simulink model "NE39bus2_PQ"  (R2023b)
settings: Solver=ode23tb  StartTime=0.0  StopTime=120  MaxStep=1/60  RelTol=1e-2  AbsTol=1e-1  EnableMultiTasking=on
PreLoadFcn:
  | NE39bus_data;
  | PSSMODEL=1;
  | LPSS=0;
  | WAPSS=0;
  | WAPSS2=0;
values from neighbouring files (symbols this model uses):
  AVR_Data = [     0.01  200    0.015   10    1    1.03    -5    5 ... (first row only)    [NE39bus_data.m]
  line = [     1	2	0.0035	0.0411	0.6987	0	100	345 ... (first row only)    [NE39bus_data.m]
  mac_con = [ ... (first row only)    [NE39bus_data.m]
  MB = [1   0.2 30   1.25 40    12 160]    [NE39bus_data.m]
  Ns = 120*60/(2)    (= 3600)    [NE39bus_data.m]
  p0 = [1000 520.81 650 632 508 650 560 540 830 250]'./1000    [NE39bus_data.m]
  s = 10    [NE39bus_data.m]
undefined symbols (not defined in the file or in its folder): D1, Delta, Pn
libraries: spsThreePhaseVIMeasurementLib x56, spsThreePhasePISectionLineLib x38, spsGenericPowerSystemStabilizerLib x20, spsThreePhaseParallelRLCLoadLib x19, spsThreePhaseTransformerTwoWindingsLib x16, spsSynchronousMachinepuStandardLib x10, spsExcitationSystemLib x10, spsMultiBandPowerSystemStabilizerLib x10, spsSteamTurbineandGovernorLib x10, spsLoadFlowBusLib x10, powerlib_extras x4, spsThreePhaseDynamicLoadLib x4
(part 4 of 5)

== system NE39bus2_PQ/G8/M8: Turbine & Regulators ==
  note: M8
  m8 : Inport
  Pref8 : Inport  Port=2
  Vref8 : Inport  Port=3
  PSS8 : Inport  Port=4
  Bus Selector : BusSelector  OutputSignals="Mechanical.Rotor speed  wm  (pu),Mechanical.Rotor angle deviation  d_theta (rad),Mechanical.Electrical power  Pe (pu),Mechanical.Rotor speed deviation  dw (pu),Mechanical.Rotor mechanical angle  theta (deg),dq0 components.Stator voltage  vd (pu),dq0 components.Stator voltage  vq (pu),Output reactive power  Qeo (pu)"
  Delta Pa PSS 8 : spsGenericPowerSystemStabilizerLib/Generic Power System Stabilizer  Tsensor=15e-3  K=2.5*1.25  Twashout=1  Tleadlag1=[60e-3 1]  Tleadlag2=[0 0]  VSlimits=[-0.15 0.15]  Vinit=0  Plot_On=off  MagdB_On=on  FreqRange=logspace(-2,2,500)
      settings: LibrarySourceBlock=|
      | sps_lib/Electrical Machines/Synchronous Machine Control/Generic
      | Power System Stabilizer
  Delta w PSS (Kundur) 8 : spsGenericPowerSystemStabilizerLib/Generic Power System Stabilizer  Tsensor=15e-3  K=30  Twashout=10  Tleadlag1=[50e-3 20e-3]  Tleadlag2=[3 5.4]  VSlimits=[-0.15 0.15]  Vinit=0  Plot_On=off  MagdB_On=on  FreqRange=logspace(-2,2,500)
      settings: LibrarySourceBlock=|
      | sps_lib/Electrical Machines/Synchronous Machine Control/Generic
      | Power System Stabilizer
  EXCITATION8 : spsExcitationSystemLib/Excitation System  tr=AVR_Data(8,1)  reg=[ AVR_Data(8,2:3) ]  exc=[ 1, 0 ]  tgr=[ AVR_Data(8,4:5)]  damp=[ 0, 0 ]  sat=[ 0, 0 ]  lim="[ AVR_Data(8,7:8)  0 ]"  v0=[1,1.90805]
      settings: LibrarySourceBlock=sps_lib/Electrical Machines/Synchronous Machine Control/Excitation System
  MB-PSS8 : spsMultiBandPowerSystemStabilizerLib/Multi-Band Power System Stabilizer  OperationMode=Simplified settings  Kg=MB(1)  GL=[MB(2) MB(3)]  GI=[MB(4) MB(5)]  GH=[MB(6) MB(7)]  GLd=[66 66 9.4]  TcLF=[1.667 2 0 0 0 0 2 2.4 0 0 0 0 1 1]  GId=[66 66 47.6]  TcIF=[1 1 0.25 0.3 0 0 1 1 0.3 0.36 0 0 0 0]  GHd=[66 66 233]  TcHF="[0.01 0.012 0 0 0 0  0.012 0.0144 0 0 0 0 1 1]"  LIM=[.075 .15 .15 .15]  Plot_On=off  MagdB_On=off  FreqRange=logspace(-2,2,500)
      settings: LibrarySourceBlock=|
      | sps_lib/Electrical Machines/Synchronous Machine Control/Multi-Band
      | Power System Stabilizer
  Multiport Switch2 : MultiPortSwitch  Inputs=4  SaturateOnIntegerOverflow=off
  PSS model1 : Constant  Value=0
  PSS model2 : Constant
  Real-Imag to Complex1 : RealImagToComplex
  STG8 : spsSteamTurbineandGovernorLib/Steam Turbine and Governor  gentype=Tandem-compound (single mass)  reg1="[ 1  0.05    0 ]"  reg2="[ 0.001  0.15 ]"  reg3="[ -0.1  0.1  0  4.496 ]"  N=Ns  turb1="[ 0  10   3.3   0.5   ]"  turb2="[   0   0.36    0.36   0.28   ]"  HA="[ 0.046  1.430  1.465   0.192 ]"  KA="[ 90.44  53.88  64.59   62.94  ]"  DA="[ 0.0115  0.3575  0.3663   0.0137  ]"  ini1=0.54  ini2=[0.779316,-31.4247]
      settings: LibrarySourceBlock=|
      | sps_lib/Electrical Machines/Synchronous Machine Control/Steam Turbine
      | and Governor
  Sum1 : Sum  Inputs=-+  InputSameDT=on  SaturateOnIntegerOverflow=on  OutDataTypeStr=Inherit: Same as first input
  Sum2 : Sum  InputSameDT=on  SaturateOnIntegerOverflow=on  OutDataTypeStr=Inherit: Same as first input
  Terminator3 : Terminator
  Terminator4 : Terminator
  Terminator5 : Terminator
  wref8 : Constant
  Pm8 : Outport  InitialOutput=0
  Vf8 : Outport  Port=2  InitialOutput=0
  tag scope: EFD8=global, Pa8=global, Pe8=global, Q8=global, Vt8=global, d_theta8=global, pss8=global, theta8=global, w8=global
  wires:
  Bus Selector/7 -> EXCITATION8/3, Real-Imag to Complex1/2  "<Stator voltage  vq (pu)>"
  wref8/1 -> STG8/1
  Pref8/1 -> STG8/2
  m8/1 -> Bus Selector/1
  Vref8/1 -> EXCITATION8/1
  EXCITATION8/1 -> Vf8/1, [EFD8]
  Real-Imag to Complex1/1 -> [Vt8]
  Bus Selector/5 -> [theta8]  "<Rotor mechanical angle  theta (deg)>"
  Bus Selector/6 -> EXCITATION8/2, Real-Imag to Complex1/1  "<Stator voltage  vd (pu)>"
  STG8/3 -> Terminator3/1
  STG8/4 -> Sum1/2, Pm8/1
  STG8/2 -> Terminator4/1
  STG8/1 -> Terminator5/1
  Bus Selector/1 -> [w8], STG8/3  "<Rotor speed  wm  (pu)>"
  Bus Selector/2 -> STG8/4, [d_theta8]  "<Rotor angle deviation  d_theta (rad)>"
  Bus Selector/3 -> Sum1/1, [Pe8]  "<Electrical power  Pe (pu)>"
  Bus Selector/4 -> MB-PSS8/1, Delta w PSS (Kundur) 8/1  "<Rotor speed deviation  dw (pu)>"
  Bus Selector/8 -> [Q8]  "<Output reactive power  Qeo (pu)>"
  Sum1/1 -> [Pa8], Delta Pa PSS 8/1  "Pm-Pe"
  Sum2/1 -> Multiport Switch2/1
  PSS model2/1 -> Sum2/2
  Delta Pa PSS 8/1 -> Multiport Switch2/5
  Delta w PSS (Kundur) 8/1 -> Multiport Switch2/4
  MB-PSS8/1 -> Multiport Switch2/3
  PSS model1/1 -> Multiport Switch2/2
  Multiport Switch2/1 -> EXCITATION8/4, [pss8]
  PSS8/1 -> Sum2/1

== system NE39bus2_PQ/G9/M9: Turbine & Regulators  ==
  note: M9
  m9 : Inport
  Pref9 : Inport  Port=2
  Vref9 : Inport  Port=3
  PSS9 : Inport  Port=4
  Bus Selector : BusSelector  OutputSignals="Mechanical.Rotor speed  wm  (pu),Mechanical.Rotor angle deviation  d_theta (rad),Mechanical.Electrical power  Pe (pu),Mechanical.Rotor speed deviation  dw (pu),Mechanical.Rotor mechanical angle  theta (deg),dq0 components.Stator voltage  vd (pu),dq0 components.Stator voltage  vq (pu),Output reactive power  Qeo (pu)"
  Delta Pa PSS 9 : spsGenericPowerSystemStabilizerLib/Generic Power System Stabilizer  Tsensor=15e-3  K=2.5*1.25  Twashout=1  Tleadlag1=[60e-3 1]  Tleadlag2=[0 0]  VSlimits=[-0.15 0.15]  Vinit=0  Plot_On=off  MagdB_On=on  FreqRange=logspace(-2,2,500)
      settings: LibrarySourceBlock=|
      | sps_lib/Electrical Machines/Synchronous Machine Control/Generic
      | Power System Stabilizer
  Delta w PSS (Kundur) 9 : spsGenericPowerSystemStabilizerLib/Generic Power System Stabilizer  Tsensor=15e-3  K=30  Twashout=10  Tleadlag1=[50e-3 20e-3]  Tleadlag2=[3 5.4]  VSlimits=[-0.15 0.15]  Vinit=0  Plot_On=off  MagdB_On=on  FreqRange=logspace(-2,2,500)
      settings: LibrarySourceBlock=|
      | sps_lib/Electrical Machines/Synchronous Machine Control/Generic
      | Power System Stabilizer
  EXCITATION9 : spsExcitationSystemLib/Excitation System  tr=AVR_Data(9,1)  reg=[ AVR_Data(9,2:3) ]  exc=[ 1, 0 ]  tgr=[ AVR_Data(9,4:5)]  damp=[ 0, 0 ]  sat=[ 0, 0 ]  lim="[ AVR_Data(9,7:8)  0 ]"  v0=[1,2.08155]
      settings: LibrarySourceBlock=sps_lib/Electrical Machines/Synchronous Machine Control/Excitation System
  MB-PSS9 : spsMultiBandPowerSystemStabilizerLib/Multi-Band Power System Stabilizer  OperationMode=Simplified settings  Kg=MB(1)  GL=[MB(2) MB(3)]  GI=[MB(4) MB(5)]  GH=[MB(6) MB(7)]  GLd=[66 66 9.4]  TcLF=[1.667 2 0 0 0 0 2 2.4 0 0 0 0 1 1]  GId=[66 66 47.6]  TcIF=[1 1 0.25 0.3 0 0 1 1 0.3 0.36 0 0 0 0]  GHd=[66 66 233]  TcHF="[0.01 0.012 0 0 0 0  0.012 0.0144 0 0 0 0 1 1]"  LIM=[.075 .15 .15 .15]  Plot_On=off  MagdB_On=off  FreqRange=logspace(-2,2,500)
      settings: LibrarySourceBlock=|
      | sps_lib/Electrical Machines/Synchronous Machine Control/Multi-Band
      | Power System Stabilizer
  Multiport Switch1 : MultiPortSwitch  Inputs=4  SaturateOnIntegerOverflow=off
  PSS model3 : Constant  Value=0
  PSS model4 : Constant
  Real-Imag to Complex1 : RealImagToComplex
  STG9 : spsSteamTurbineandGovernorLib/Steam Turbine and Governor  gentype=Tandem-compound (single mass)  reg1="[ 1  0.05    0 ]"  reg2="[ 0.001  0.15 ]"  reg3="[ -0.1  0.1  0  4.496 ]"  N=Ns  turb1="[ 0  10   3.3   0.5   ]"  turb2="[   0   0.36    0.36   0.28   ]"  HA="[ 0.046  1.430  1.465   0.192 ]"  KA="[ 90.44  53.88  64.59   62.94  ]"  DA="[ 0.0115  0.3575  0.3663   0.0137  ]"  ini1=0.83  ini2=[0.779316,-31.4247]
      settings: LibrarySourceBlock=|
      | sps_lib/Electrical Machines/Synchronous Machine Control/Steam Turbine
      | and Governor
  Sum2 : Sum  InputSameDT=on  SaturateOnIntegerOverflow=on  OutDataTypeStr=Inherit: Same as first input
  Sum3 : Sum  Inputs=-+  InputSameDT=on  SaturateOnIntegerOverflow=on  OutDataTypeStr=Inherit: Same as first input
  Terminator3 : Terminator
  Terminator4 : Terminator
  Terminator5 : Terminator
  wref9 : Constant
  Pm9 : Outport  InitialOutput=0
  Vf9 : Outport  Port=2  InitialOutput=0
  tag scope: EFD9=global, Pa9=global, Pe9=global, Q9=global, Vt9=global, d_theta9=global, pss9=global, theta9=global, w9=global
  wires:
  Bus Selector/7 -> EXCITATION9/3, Real-Imag to Complex1/2  "<Stator voltage  vq (pu)>"
  wref9/1 -> STG9/1
  Pref9/1 -> STG9/2
  m9/1 -> Bus Selector/1
  Vref9/1 -> EXCITATION9/1
  EXCITATION9/1 -> Vf9/1, [EFD9]
  Real-Imag to Complex1/1 -> [Vt9]
  Bus Selector/5 -> [theta9]  "<Rotor mechanical angle  theta (deg)>"
  Bus Selector/6 -> EXCITATION9/2, Real-Imag to Complex1/1  "<Stator voltage  vd (pu)>"
  STG9/3 -> Terminator3/1
  STG9/4 -> Sum3/2, Pm9/1
  STG9/2 -> Terminator4/1
  STG9/1 -> Terminator5/1
  Bus Selector/1 -> [w9], STG9/3  "<Rotor speed  wm  (pu)>"
  Bus Selector/2 -> STG9/4, [d_theta9]  "<Rotor angle deviation  d_theta (rad)>"
  Bus Selector/3 -> Sum3/1, [Pe9]  "<Electrical power  Pe (pu)>"
  Bus Selector/4 -> Delta w PSS (Kundur) 9/1, MB-PSS9/1  "<Rotor speed deviation  dw (pu)>"
  Bus Selector/8 -> [Q9]  "<Output reactive power  Qeo (pu)>"
  Sum3/1 -> [Pa9], Delta Pa PSS 9/1  "Pm-Pe"
  Sum2/1 -> Multiport Switch1/1
  PSS model4/1 -> Sum2/2
  Delta Pa PSS 9/1 -> Multiport Switch1/5
  Delta w PSS (Kundur) 9/1 -> Multiport Switch1/4
  MB-PSS9/1 -> Multiport Switch1/3
  PSS model3/1 -> Multiport Switch1/2
  Multiport Switch1/1 -> [pss9], EXCITATION9/4
  PSS9/1 -> Sum2/1

== matlab function NE39bus2_PQ/DCLoad3/DC Composite Model/DC ==
  data: V_pu input; P_out output; Q_out output; t input; ups_state output; cool_stall output; P_it_out output; P_ai_pu input; P_cool_out output; Pdc_MW input
function [P_out, Q_out, ups_state, cool_stall, P_it_out, P_cool_out] = ...
    datacenter_motorE(V_pu, t, P_ai_pu, Pdc_MW)
%#codegen
% =========================================================================
% WECC CLM Extension: Data Center Load Model (Motor E)
% Scalable from 100 MW to 500 MW
% =========================================================================
% Inputs:  V_pu    = per-unit voltage at load bus
%          t       = simulation time
%          P_ai_pu = AI workload demand (0-1 pu)
%          Pdc_MW  = data center rated power in MW (100 to 500)
%
% Outputs: P_out (W), Q_out (VAR)
%          ups_state, cool_stall, P_it_out, P_cool_out
%
% Block sample time = 0.001
% =========================================================================

dt = 0.001;

% ===== DATA CENTER SIZING =====
Pdc = double(Pdc_MW(1)) * 1e6;    % convert MW to W

% ===== SUB-COMPONENT FRACTIONS =====
% Based on industry data:
% IT load (servers/GPUs): 55-65% -> 60%
% Cooling (chillers/CRAH): 25-35% -> 30%
% Auxiliary (lighting/office/network): 8-12% -> 10%
Fit_max  = 0.60;
Fcool    = 0.30;
Faux     = 0.10;

% ===== UPS PARAMETERS =====
% Large DC UPS: tighter voltage tolerance, faster transfer
V_ups_trip    = 0.90;    % static transfer switch threshold
V_ups_return  = 0.95;    % return to grid threshold
T_ups_battery = 30.0;    % battery hold-up time (s)
T_diesel_start = 12.0;   % diesel generator start time (s)
T_ups_transfer = 0.004;  % static switch transfer time (s)
PF_it = 0.95;

% ===== COOLING PARAMETERS =====
% Industrial chillers: higher inertia, different stall characteristics
Rstall_c = 0.10;     Xstall_c = 0.12;
Vstall_c = 0.55;     % industrial compressors stall lower than residential
Tstall_c = 0.05;     % stall confirmation delay
Vrst_c   = 0.90;     Trst_c = 2.0;   % slower restart (large chillers)
TTH_c    = 60;        % higher thermal mass (industrial)
th1_c    = 1.6;       th2_c = 2.8;    % wider thermal margin
PF_cool  = 0.85;

% ===== VFD COOLING FRACTION =====
% Modern DCs use VFDs on some chillers (don't stall, ride through)
Fvfd = 0.40;    % 40% of cooling on VFDs (constant power during fault)

% ===== PERSISTENT STATE =====
persistent ups_mode batt_timer diesel_timer transfer_cnt
persistent is_cool_stalled cool_stall_cnt cool_rst_cnt
persistent theta_cool fth_cool
persistent P_it_before_fault
persistent rebound_active rebound_timer
persistent init_done

if isempty(init_done)
    ups_mode          = 0;
    batt_timer        = 0;
    diesel_timer      = 0;
    transfer_cnt      = 0;
    is_cool_stalled   = false;
    cool_stall_cnt    = 0;
    cool_rst_cnt      = 0;
    theta_cool        = 0;
    fth_cool          = 1;
    P_it_before_fault = 0;
    rebound_active    = false;
    rebound_timer     = 0;
    init_done         = true;
end

% Soft start
if t < 1.0
    ramp = t / 1.0;
    P_out = Pdc * 0.7 * ramp;
    Q_out = Pdc * 0.25 * ramp;
    ups_state  = 0;
    cool_stall = 0;
    P_it_out   = Fit_max * Pdc * 0.9 * ramp;
    P_cool_out = Fcool * Pdc * ramp;
    return;
end

V = double(V_pu(1));
if V < 0.01
    V = 0.01;
end
if V > 1.5
    V = 1.5;
end

P_ai = double(P_ai_pu(1));
if P_ai < 0.05
    P_ai = 0.05;
end
if P_ai > 1.0
    P_ai = 1.0;
end

% =========================================================
% COMPONENT 1: IT LOAD WITH UPS + AI WORKLOAD
% =========================================================
P_it_demand = Fit_max * Pdc * P_ai;
Q_it_demand = P_it_demand * tan(acos(PF_it));

P_it = 0;
Q_it = 0;

if ups_mode == 0
    % GRID-CONNECTED: IT load on grid, scaled by workload
    P_it_before_fault = P_it_demand;
    
    if V < V_ups_trip
        ups_mode = 1;
        batt_timer = 0;
        diesel_timer = 0;
        transfer_cnt = 0;
    end
    
    P_it = P_it_demand;
    Q_it = Q_it_demand;
    
elseif ups_mode == 1
    % UPS BATTERY MODE: IT load invisible to grid
    batt_timer = batt_timer + dt;
    diesel_timer = diesel_timer + dt;
    transfer_cnt = transfer_cnt + dt;
    
    if transfer_cnt < T_ups_transfer
        % During transfer: partial load visible
        P_it = P_it_before_fault * 0.3;
        Q_it = Q_it_demand * 0.3;
    else
        % Fully on battery: zero grid draw
        P_it = 0;
        Q_it = 0;
    end
    
    if V >= V_ups_return
        % Voltage recovered: LOAD REBOUND
        ups_mode = 0;
        rebound_active = true;
        rebound_timer = 0;
        batt_timer = 0;
    elseif diesel_timer >= T_diesel_start
        ups_mode = 2;
    elseif batt_timer >= T_ups_battery
        ups_mode = 0;  % forced return
        rebound_active = true;
        rebound_timer = 0;
    end
    
elseif ups_mode == 2
    % DIESEL BACKUP: permanently off grid
    P_it = 0;
    Q_it = 0;
end

% LOAD REBOUND: IT load returns to grid with inrush
% Causes a secondary voltage dip
if rebound_active
    rebound_timer = rebound_timer + dt;
    rebound_duration = 0.5;  % 500ms rebound transient
    
    if rebound_timer < rebound_duration
        % During rebound: 120% of pre-fault load (inrush)
        rebound_factor = 1.2 - 0.2 * (rebound_timer / rebound_duration);
        P_it = P_it * rebound_factor;
        Q_it = Q_it * rebound_factor * 1.5;  % higher Q during rebound
    else
        rebound_active = false;
    end
end

% =========================================================
% COMPONENT 2: COOLING LOAD (split: motor + VFD)
% =========================================================

Zstall_sq = Rstall_c * Rstall_c + Xstall_c * Xstall_c;
Gstall_cool = Rstall_c / Zstall_sq;
Bstall_cool = Xstall_c / Zstall_sq;

% Cooling demand proportional to IT workload
cool_scale = 0.4 + 0.6 * P_ai;  % 60-100% cooling

P_cool_base = Fcool * Pdc * cool_scale;
Q_cool_base = P_cool_base * tan(acos(PF_cool));

% --- Motor-driven portion (1-Fvfd): can stall ---
P_motor_rated = (1.0 - Fvfd) * P_cool_base;
Q_motor_rated = (1.0 - Fvfd) * Q_cool_base;

P_motor_stall = Gstall_cool * V * V * (1.0 - Fvfd) * Fcool * Pdc;
Q_motor_stall = -Bstall_cool * V * V * (1.0 - Fvfd) * Fcool * Pdc;

% Stall logic (motor portion only)
if ~is_cool_stalled
    if V < Vstall_c
        cool_stall_cnt = cool_stall_cnt + dt;
        if cool_stall_cnt >= Tstall_c
            is_cool_stalled = true;
            cool_stall_cnt = 0;
        end
    else
        cool_stall_cnt = 0;
    end
else
    if V >= Vrst_c
        cool_rst_cnt = cool_rst_cnt + dt;
        if cool_rst_cnt >= Trst_c
            is_cool_stalled = false;
            cool_rst_cnt = 0;
            theta_cool = 0;
        end
    else
        cool_rst_cnt = 0;
    end
end

% Thermal relay
if is_cool_stalled
    I_sq = V * V / Zstall_sq;
    theta_cool = theta_cool + (I_sq * Rstall_c - theta_cool) / TTH_c * dt;
    if theta_cool < 0
        theta_cool = 0;
    end
    if theta_cool >= th2_c
        fth_cool = 0;
    elseif theta_cool >= th1_c
        fth_cool = 1.0 - (theta_cool - th1_c) / (th2_c - th1_c);
        if fth_cool < 0
            fth_cool = 0;
        end
    else
        fth_cool = 1.0;
    end
else
    if theta_cool > 0.001
        theta_cool = theta_cool * (1.0 - dt / TTH_c);
    else
        theta_cool = 0;
    end
    fth_cool = 1.0;
end

% Motor cooling output
if is_cool_stalled
    P_motor = P_motor_stall * fth_cool;
    Q_motor = Q_motor_stall * fth_cool;
else
    P_motor = P_motor_rated * V * V;
    Q_motor = Q_motor_rated * V * V;
end

% --- VFD portion (Fvfd): rides through, constant power ---
% VFDs maintain constant power down to ~0.5 pu voltage
if V >= 0.5
    P_vfd = Fvfd * P_cool_base;
    Q_vfd = Fvfd * Q_cool_base * 0.5;  % VFDs have lower Q
elseif V >= 0.3
    % Linear reduction below 0.5
    vfd_frac = (V - 0.3) / 0.2;
    P_vfd = Fvfd * P_cool_base * vfd_frac;
    Q_vfd = Fvfd * Q_cool_base * 0.5 * vfd_frac;
else
    P_vfd = 0;
    Q_vfd = 0;
end

P_cool = P_motor + P_vfd;
Q_cool = Q_motor + Q_vfd;

% =========================================================
% COMPONENT 3: AUXILIARY (constant impedance)
% =========================================================
P_aux = Faux * Pdc * V * V;
Q_aux = Faux * Pdc * 0.15 * V * V;

% =========================================================
% TOTAL DATA CENTER OUTPUT
% =========================================================
P_out = P_it + P_cool + P_aux;
Q_out = Q_it + Q_cool + Q_aux;

if P_out < 0
    P_out = 0;
end

ups_state = double(ups_mode);
if is_cool_stalled
    cool_stall = 1.0;
else
    cool_stall = 0.0;
end
P_it_out = P_it;
P_cool_out = P_cool;

end

== matlab function NE39bus2_PQ/DCLoad1/DC Composite Model/AI Workload Generator ==
  data: t input; mode input; P_ai_pu output; workload_label output
function [P_ai_pu, workload_label] = ai_workload(t, mode)
%#codegen
% AI GPU Workload Profile Generator
% mode: 1=Training, 2=Inference, 3=Idle
% Output: P_ai_pu (0 to 1), workload_label

workload_label = double(mode);

if mode == 1
    % TRAINING: sustained high with checkpoint dips
    base_power = 0.3;
    checkpoint_interval = 60.0;
    checkpoint_duration = 2.0;
    checkpoint_dip = 0.40;
    comm_period = 1.2;
    comm_amplitude = 0.6;
    
    time_in_cycle = mod(t, checkpoint_interval);
    if time_in_cycle < checkpoint_duration
        P_ai_pu = checkpoint_dip;
    else
        oscillation = comm_amplitude * sin(2.0 * 3.14159 * t / comm_period);
        P_ai_pu = base_power + oscillation;
    end
    
elseif mode == 2
    % INFERENCE: bursty multi-frequency
    base_power = 0.15;
    burst1 = 0.25 * sin(2.0 * 3.14159 * t / 5.0);
    burst2 = 0.15 * sin(2.0 * 3.14159 * t / 1.3);
    burst3 = 0.10 * sin(2.0 * 3.14159 * t / 0.4);
    
    if t < 2.0
        diurnal = 0.5 + 0.5 * (t / 2.0);
    else
        diurnal = 1.0;
    end
    
    P_ai_pu = (base_power + burst1 + burst2 + burst3) * diurnal;
    
elseif mode == 3
    % IDLE
    P_ai_pu = 0.15;
else
    P_ai_pu = 0.5;
end

if P_ai_pu < 0.05
    P_ai_pu = 0.05;
end
if P_ai_pu > 1.0
    P_ai_pu = 1.0;
end

end

== matlab function NE39bus2_PQ/DCLoad1/DC Composite Model/DC ==
  data: V_pu input; P_out output; Q_out output; t input; ups_state output; cool_stall output; P_it_out output; P_ai_pu input; P_cool_out output; Pdc_MW input
function [P_out, Q_out, ups_state, cool_stall, P_it_out, P_cool_out] = ...
    datacenter_motorE(V_pu, t, P_ai_pu, Pdc_MW)
%#codegen
% =========================================================================
% WECC CLM Extension: Data Center Load Model (Motor E)
% Scalable from 100 MW to 500 MW
% =========================================================================
% Inputs:  V_pu    = per-unit voltage at load bus
%          t       = simulation time
%          P_ai_pu = AI workload demand (0-1 pu)
%          Pdc_MW  = data center rated power in MW (100 to 500)
%
% Outputs: P_out (W), Q_out (VAR)
%          ups_state, cool_stall, P_it_out, P_cool_out
%
% Block sample time = 0.001
% =========================================================================

dt = 0.001;

% ===== DATA CENTER SIZING =====
Pdc = double(Pdc_MW(1)) * 1e6;    % convert MW to W

% ===== SUB-COMPONENT FRACTIONS =====
% Based on industry data:
% IT load (servers/GPUs): 55-65% -> 60%
% Cooling (chillers/CRAH): 25-35% -> 30%
% Auxiliary (lighting/office/network): 8-12% -> 10%
Fit_max  = 0.60;
Fcool    = 0.30;
Faux     = 0.10;

% ===== UPS PARAMETERS =====
% Large DC UPS: tighter voltage tolerance, faster transfer
V_ups_trip    = 0.90;    % static transfer switch threshold
V_ups_return  = 0.95;    % return to grid threshold
T_ups_battery = 30.0;    % battery hold-up time (s)
T_diesel_start = 12.0;   % diesel generator start time (s)
T_ups_transfer = 0.004;  % static switch transfer time (s)
PF_it = 0.95;

% ===== COOLING PARAMETERS =====
% Industrial chillers: higher inertia, different stall characteristics
Rstall_c = 0.10;     Xstall_c = 0.12;
Vstall_c = 0.55;     % industrial compressors stall lower than residential
Tstall_c = 0.05;     % stall confirmation delay
Vrst_c   = 0.90;     Trst_c = 2.0;   % slower restart (large chillers)
TTH_c    = 60;        % higher thermal mass (industrial)
th1_c    = 1.6;       th2_c = 2.8;    % wider thermal margin
PF_cool  = 0.85;

% ===== VFD COOLING FRACTION =====
% Modern DCs use VFDs on some chillers (don't stall, ride through)
Fvfd = 0.40;    % 40% of cooling on VFDs (constant power during fault)

% ===== PERSISTENT STATE =====
persistent ups_mode batt_timer diesel_timer transfer_cnt
persistent is_cool_stalled cool_stall_cnt cool_rst_cnt
persistent theta_cool fth_cool
persistent P_it_before_fault
persistent rebound_active rebound_timer
persistent init_done

if isempty(init_done)
    ups_mode          = 0;
    batt_timer        = 0;
    diesel_timer      = 0;
    transfer_cnt      = 0;
    is_cool_stalled   = false;
    cool_stall_cnt    = 0;
    cool_rst_cnt      = 0;
    theta_cool        = 0;
    fth_cool          = 1;
    P_it_before_fault = 0;
    rebound_active    = false;
    rebound_timer     = 0;
    init_done         = true;
end

% Soft start
if t < 1.0
    ramp = t / 1.0;
    P_out = Pdc * 0.7 * ramp;
    Q_out = Pdc * 0.25 * ramp;
    ups_state  = 0;
    cool_stall = 0;
    P_it_out   = Fit_max * Pdc * 0.9 * ramp;
    P_cool_out = Fcool * Pdc * ramp;
    return;
end

V = double(V_pu(1));
if V < 0.01
    V = 0.01;
end
if V > 1.5
    V = 1.5;
end

P_ai = double(P_ai_pu(1));
if P_ai < 0.05
    P_ai = 0.05;
end
if P_ai > 1.0
    P_ai = 1.0;
end

% =========================================================
% COMPONENT 1: IT LOAD WITH UPS + AI WORKLOAD
% =========================================================
P_it_demand = Fit_max * Pdc * P_ai;
Q_it_demand = P_it_demand * tan(acos(PF_it));

P_it = 0;
Q_it = 0;

if ups_mode == 0
    % GRID-CONNECTED: IT load on grid, scaled by workload
    P_it_before_fault = P_it_demand;
    
    if V < V_ups_trip
        ups_mode = 1;
        batt_timer = 0;
        diesel_timer = 0;
        transfer_cnt = 0;
    end
    
    P_it = P_it_demand;
    Q_it = Q_it_demand;
    
elseif ups_mode == 1
    % UPS BATTERY MODE: IT load invisible to grid
    batt_timer = batt_timer + dt;
    diesel_timer = diesel_timer + dt;
    transfer_cnt = transfer_cnt + dt;
    
    if transfer_cnt < T_ups_transfer
        % During transfer: partial load visible
        P_it = P_it_before_fault * 0.3;
        Q_it = Q_it_demand * 0.3;
    else
        % Fully on battery: zero grid draw
        P_it = 0;
        Q_it = 0;
    end
    
    if V >= V_ups_return
        % Voltage recovered: LOAD REBOUND
        ups_mode = 0;
        rebound_active = true;
        rebound_timer = 0;
        batt_timer = 0;
    elseif diesel_timer >= T_diesel_start
        ups_mode = 2;
    elseif batt_timer >= T_ups_battery
        ups_mode = 0;  % forced return
        rebound_active = true;
        rebound_timer = 0;
    end
    
elseif ups_mode == 2
    % DIESEL BACKUP: permanently off grid
    P_it = 0;
    Q_it = 0;
end

% LOAD REBOUND: IT load returns to grid with inrush
% Causes a secondary voltage dip
if rebound_active
    rebound_timer = rebound_timer + dt;
    rebound_duration = 0.5;  % 500ms rebound transient
    
    if rebound_timer < rebound_duration
        % During rebound: 120% of pre-fault load (inrush)
        rebound_factor = 1.2 - 0.2 * (rebound_timer / rebound_duration);
        P_it = P_it * rebound_factor;
        Q_it = Q_it * rebound_factor * 1.5;  % higher Q during rebound
    else
        rebound_active = false;
    end
end

% =========================================================
% COMPONENT 2: COOLING LOAD (split: motor + VFD)
% =========================================================

Zstall_sq = Rstall_c * Rstall_c + Xstall_c * Xstall_c;
Gstall_cool = Rstall_c / Zstall_sq;
Bstall_cool = Xstall_c / Zstall_sq;

% Cooling demand proportional to IT workload
cool_scale = 0.4 + 0.6 * P_ai;  % 60-100% cooling

P_cool_base = Fcool * Pdc * cool_scale;
Q_cool_base = P_cool_base * tan(acos(PF_cool));

% --- Motor-driven portion (1-Fvfd): can stall ---
P_motor_rated = (1.0 - Fvfd) * P_cool_base;
Q_motor_rated = (1.0 - Fvfd) * Q_cool_base;

P_motor_stall = Gstall_cool * V * V * (1.0 - Fvfd) * Fcool * Pdc;
Q_motor_stall = -Bstall_cool * V * V * (1.0 - Fvfd) * Fcool * Pdc;

% Stall logic (motor portion only)
if ~is_cool_stalled
    if V < Vstall_c
        cool_stall_cnt = cool_stall_cnt + dt;
        if cool_stall_cnt >= Tstall_c
            is_cool_stalled = true;
            cool_stall_cnt = 0;
        end
    else
        cool_stall_cnt = 0;
    end
else
    if V >= Vrst_c
        cool_rst_cnt = cool_rst_cnt + dt;
        if cool_rst_cnt >= Trst_c
            is_cool_stalled = false;
            cool_rst_cnt = 0;
            theta_cool = 0;
        end
    else
        cool_rst_cnt = 0;
    end
end

% Thermal relay
if is_cool_stalled
    I_sq = V * V / Zstall_sq;
    theta_cool = theta_cool + (I_sq * Rstall_c - theta_cool) / TTH_c * dt;
    if theta_cool < 0
        theta_cool = 0;
    end
    if theta_cool >= th2_c
        fth_cool = 0;
    elseif theta_cool >= th1_c
        fth_cool = 1.0 - (theta_cool - th1_c) / (th2_c - th1_c);
        if fth_cool < 0
            fth_cool = 0;
        end
    else
        fth_cool = 1.0;
    end
else
    if theta_cool > 0.001
        theta_cool = theta_cool * (1.0 - dt / TTH_c);
    else
        theta_cool = 0;
    end
    fth_cool = 1.0;
end

% Motor cooling output
if is_cool_stalled
    P_motor = P_motor_stall * fth_cool;
    Q_motor = Q_motor_stall * fth_cool;
else
    P_motor = P_motor_rated * V * V;
    Q_motor = Q_motor_rated * V * V;
end

% --- VFD portion (Fvfd): rides through, constant power ---
% VFDs maintain constant power down to ~0.5 pu voltage
if V >= 0.5
    P_vfd = Fvfd * P_cool_base;
    Q_vfd = Fvfd * Q_cool_base * 0.5;  % VFDs have lower Q
elseif V >= 0.3
    % Linear reduction below 0.5
    vfd_frac = (V - 0.3) / 0.2;
    P_vfd = Fvfd * P_cool_base * vfd_frac;
    Q_vfd = Fvfd * Q_cool_base * 0.5 * vfd_frac;
else
    P_vfd = 0;
    Q_vfd = 0;
end

P_cool = P_motor + P_vfd;
Q_cool = Q_motor + Q_vfd;

% =========================================================
% COMPONENT 3: AUXILIARY (constant impedance)
% =========================================================
P_aux = Faux * Pdc * V * V;
Q_aux = Faux * Pdc * 0.15 * V * V;

% =========================================================
% TOTAL DATA CENTER OUTPUT
% =========================================================
P_out = P_it + P_cool + P_aux;
Q_out = Q_it + Q_cool + Q_aux;

if P_out < 0
    P_out = 0;
end

ups_state = double(ups_mode);
if is_cool_stalled
    cool_stall = 1.0;
else
    cool_stall = 0.0;
end
P_it_out = P_it;
P_cool_out = P_cool;

end

== matlab function NE39bus2_PQ/DCLoad2/DC Composite Model/AI Workload Generator ==
  data: t input; mode input; P_ai_pu output; workload_label output
function [P_ai_pu, workload_label] = ai_workload(t, mode)
%#codegen
% AI GPU Workload Profile Generator
% mode: 1=Training, 2=Inference, 3=Idle
% Output: P_ai_pu (0 to 1), workload_label

workload_label = double(mode);

if mode == 1
    % TRAINING: sustained high with checkpoint dips
    base_power = 0.3;
    checkpoint_interval = 60.0;
    checkpoint_duration = 2.0;
    checkpoint_dip = 0.40;
    comm_period = 1.2;
    comm_amplitude = 0.6;
    
    time_in_cycle = mod(t, checkpoint_interval);
    if time_in_cycle < checkpoint_duration
        P_ai_pu = checkpoint_dip;
    else
        oscillation = comm_amplitude * sin(2.0 * 3.14159 * t / comm_period);
        P_ai_pu = base_power + oscillation;
    end
    
elseif mode == 2
    % INFERENCE: bursty multi-frequency
    base_power = 0.15;
    burst1 = 0.25 * sin(2.0 * 3.14159 * t / 5.0);
    burst2 = 0.15 * sin(2.0 * 3.14159 * t / 1.3);
    burst3 = 0.10 * sin(2.0 * 3.14159 * t / 0.4);
    
    if t < 2.0
        diurnal = 0.5 + 0.5 * (t / 2.0);
    else
        diurnal = 1.0;
    end
    
    P_ai_pu = (base_power + burst1 + burst2 + burst3) * diurnal;
    
elseif mode == 3
    % IDLE
    P_ai_pu = 0.15;
else
    P_ai_pu = 0.5;
end

if P_ai_pu < 0.05
    P_ai_pu = 0.05;
end
if P_ai_pu > 1.0
    P_ai_pu = 1.0;
end

end

== matlab function NE39bus2_PQ/DCLoad2/DC Composite Model/DC ==
  data: V_pu input; P_out output; Q_out output; t input; ups_state output; cool_stall output; P_it_out output; P_ai_pu input; P_cool_out output; Pdc_MW input
function [P_out, Q_out, ups_state, cool_stall, P_it_out, P_cool_out] = ...
    datacenter_motorE(V_pu, t, P_ai_pu, Pdc_MW)
%#codegen
% =========================================================================
% WECC CLM Extension: Data Center Load Model (Motor E)
% Scalable from 100 MW to 500 MW
% =========================================================================
% Inputs:  V_pu    = per-unit voltage at load bus
%          t       = simulation time
%          P_ai_pu = AI workload demand (0-1 pu)
%          Pdc_MW  = data center rated power in MW (100 to 500)
%
% Outputs: P_out (W), Q_out (VAR)
%          ups_state, cool_stall, P_it_out, P_cool_out
%
% Block sample time = 0.001
% =========================================================================

dt = 0.001;

% ===== DATA CENTER SIZING =====
Pdc = double(Pdc_MW(1)) * 1e6;    % convert MW to W

% ===== SUB-COMPONENT FRACTIONS =====
% Based on industry data:
% IT load (servers/GPUs): 55-65% -> 60%
% Cooling (chillers/CRAH): 25-35% -> 30%
% Auxiliary (lighting/office/network): 8-12% -> 10%
Fit_max  = 0.60;
Fcool    = 0.30;
Faux     = 0.10;

% ===== UPS PARAMETERS =====
% Large DC UPS: tighter voltage tolerance, faster transfer
V_ups_trip    = 0.90;    % static transfer switch threshold
V_ups_return  = 0.95;    % return to grid threshold
T_ups_battery = 30.0;    % battery hold-up time (s)
T_diesel_start = 12.0;   % diesel generator start time (s)
T_ups_transfer = 0.004;  % static switch transfer time (s)
PF_it = 0.95;

% ===== COOLING PARAMETERS =====
% Industrial chillers: higher inertia, different stall characteristics
Rstall_c = 0.10;     Xstall_c = 0.12;
Vstall_c = 0.55;     % industrial compressors stall lower than residential
Tstall_c = 0.05;     % stall confirmation delay
Vrst_c   = 0.90;     Trst_c = 2.0;   % slower restart (large chillers)
TTH_c    = 60;        % higher thermal mass (industrial)
th1_c    = 1.6;       th2_c = 2.8;    % wider thermal margin
PF_cool  = 0.85;

% ===== VFD COOLING FRACTION =====
% Modern DCs use VFDs on some chillers (don't stall, ride through)
Fvfd = 0.40;    % 40% of cooling on VFDs (constant power during fault)

% ===== PERSISTENT STATE =====
persistent ups_mode batt_timer diesel_timer transfer_cnt
persistent is_cool_stalled cool_stall_cnt cool_rst_cnt
persistent theta_cool fth_cool
persistent P_it_before_fault
persistent rebound_active rebound_timer
persistent init_done

if isempty(init_done)
    ups_mode          = 0;
    batt_timer        = 0;
    diesel_timer      = 0;
    transfer_cnt      = 0;
    is_cool_stalled   = false;
    cool_stall_cnt    = 0;
    cool_rst_cnt      = 0;
    theta_cool        = 0;
    fth_cool          = 1;
    P_it_before_fault = 0;
    rebound_active    = false;
    rebound_timer     = 0;
    init_done         = true;
end

% Soft start
if t < 1.0
    ramp = t / 1.0;
    P_out = Pdc * 0.7 * ramp;
    Q_out = Pdc * 0.25 * ramp;
    ups_state  = 0;
    cool_stall = 0;
    P_it_out   = Fit_max * Pdc * 0.9 * ramp;
    P_cool_out = Fcool * Pdc * ramp;
    return;
end

V = double(V_pu(1));
if V < 0.01
    V = 0.01;
end
if V > 1.5
    V = 1.5;
end

P_ai = double(P_ai_pu(1));
if P_ai < 0.05
    P_ai = 0.05;
end
if P_ai > 1.0
    P_ai = 1.0;
end

% =========================================================
% COMPONENT 1: IT LOAD WITH UPS + AI WORKLOAD
% =========================================================
P_it_demand = Fit_max * Pdc * P_ai;
Q_it_demand = P_it_demand * tan(acos(PF_it));

P_it = 0;
Q_it = 0;

if ups_mode == 0
    % GRID-CONNECTED: IT load on grid, scaled by workload
    P_it_before_fault = P_it_demand;
    
    if V < V_ups_trip
        ups_mode = 1;
        batt_timer = 0;
        diesel_timer = 0;
        transfer_cnt = 0;
    end
    
    P_it = P_it_demand;
    Q_it = Q_it_demand;
    
elseif ups_mode == 1
    % UPS BATTERY MODE: IT load invisible to grid
    batt_timer = batt_timer + dt;
    diesel_timer = diesel_timer + dt;
    transfer_cnt = transfer_cnt + dt;
    
    if transfer_cnt < T_ups_transfer
        % During transfer: partial load visible
        P_it = P_it_before_fault * 0.3;
        Q_it = Q_it_demand * 0.3;
    else
        % Fully on battery: zero grid draw
        P_it = 0;
        Q_it = 0;
    end
    
    if V >= V_ups_return
        % Voltage recovered: LOAD REBOUND
        ups_mode = 0;
        rebound_active = true;
        rebound_timer = 0;
        batt_timer = 0;
    elseif diesel_timer >= T_diesel_start
        ups_mode = 2;
    elseif batt_timer >= T_ups_battery
        ups_mode = 0;  % forced return
        rebound_active = true;
        rebound_timer = 0;
    end
    
elseif ups_mode == 2
    % DIESEL BACKUP: permanently off grid
    P_it = 0;
    Q_it = 0;
end

% LOAD REBOUND: IT load returns to grid with inrush
% Causes a secondary voltage dip
if rebound_active
    rebound_timer = rebound_timer + dt;
    rebound_duration = 0.5;  % 500ms rebound transient
    
    if rebound_timer < rebound_duration
        % During rebound: 120% of pre-fault load (inrush)
        rebound_factor = 1.2 - 0.2 * (rebound_timer / rebound_duration);
        P_it = P_it * rebound_factor;
        Q_it = Q_it * rebound_factor * 1.5;  % higher Q during rebound
    else
        rebound_active = false;
    end
end

% =========================================================
% COMPONENT 2: COOLING LOAD (split: motor + VFD)
% =========================================================

Zstall_sq = Rstall_c * Rstall_c + Xstall_c * Xstall_c;
Gstall_cool = Rstall_c / Zstall_sq;
Bstall_cool = Xstall_c / Zstall_sq;

% Cooling demand proportional to IT workload
cool_scale = 0.4 + 0.6 * P_ai;  % 60-100% cooling

P_cool_base = Fcool * Pdc * cool_scale;
Q_cool_base = P_cool_base * tan(acos(PF_cool));

% --- Motor-driven portion (1-Fvfd): can stall ---
P_motor_rated = (1.0 - Fvfd) * P_cool_base;
Q_motor_rated = (1.0 - Fvfd) * Q_cool_base;

P_motor_stall = Gstall_cool * V * V * (1.0 - Fvfd) * Fcool * Pdc;
Q_motor_stall = -Bstall_cool * V * V * (1.0 - Fvfd) * Fcool * Pdc;

% Stall logic (motor portion only)
if ~is_cool_stalled
    if V < Vstall_c
        cool_stall_cnt = cool_stall_cnt + dt;
        if cool_stall_cnt >= Tstall_c
            is_cool_stalled = true;
            cool_stall_cnt = 0;
        end
    else
        cool_stall_cnt = 0;
    end
else
    if V >= Vrst_c
        cool_rst_cnt = cool_rst_cnt + dt;
        if cool_rst_cnt >= Trst_c
            is_cool_stalled = false;
            cool_rst_cnt = 0;
            theta_cool = 0;
        end
    else
        cool_rst_cnt = 0;
    end
end

% Thermal relay
if is_cool_stalled
    I_sq = V * V / Zstall_sq;
    theta_cool = theta_cool + (I_sq * Rstall_c - theta_cool) / TTH_c * dt;
    if theta_cool < 0
        theta_cool = 0;
    end
    if theta_cool >= th2_c
        fth_cool = 0;
    elseif theta_cool >= th1_c
        fth_cool = 1.0 - (theta_cool - th1_c) / (th2_c - th1_c);
        if fth_cool < 0
            fth_cool = 0;
        end
    else
        fth_cool = 1.0;
    end
else
    if theta_cool > 0.001
        theta_cool = theta_cool * (1.0 - dt / TTH_c);
    else
        theta_cool = 0;
    end
    fth_cool = 1.0;
end

% Motor cooling output
if is_cool_stalled
    P_motor = P_motor_stall * fth_cool;
    Q_motor = Q_motor_stall * fth_cool;
else
    P_motor = P_motor_rated * V * V;
    Q_motor = Q_motor_rated * V * V;
end

% --- VFD portion (Fvfd): rides through, constant power ---
% VFDs maintain constant power down to ~0.5 pu voltage
if V >= 0.5
    P_vfd = Fvfd * P_cool_base;
    Q_vfd = Fvfd * Q_cool_base * 0.5;  % VFDs have lower Q
elseif V >= 0.3
    % Linear reduction below 0.5
    vfd_frac = (V - 0.3) / 0.2;
    P_vfd = Fvfd * P_cool_base * vfd_frac;
    Q_vfd = Fvfd * Q_cool_base * 0.5 * vfd_frac;
else
    P_vfd = 0;
    Q_vfd = 0;
end

P_cool = P_motor + P_vfd;
Q_cool = Q_motor + Q_vfd;

% =========================================================
% COMPONENT 3: AUXILIARY (constant impedance)
% =========================================================
P_aux = Faux * Pdc * V * V;
Q_aux = Faux * Pdc * 0.15 * V * V;

% =========================================================
% TOTAL DATA CENTER OUTPUT
% =========================================================
P_out = P_it + P_cool + P_aux;
Q_out = Q_it + Q_cool + Q_aux;

if P_out < 0
    P_out = 0;
end

ups_state = double(ups_mode);
if is_cool_stalled
    cool_stall = 1.0;
else
    cool_stall = 0.0;
end
P_it_out = P_it;
P_cool_out = P_cool;

end

== matlab function NE39bus2_PQ/DCLoad3/DC Composite Model/AI Workload Generator ==
  data: t input; mode input; P_ai_pu output; workload_label output
function [P_ai_pu, workload_label] = ai_workload(t, mode)
%#codegen
% AI GPU Workload Profile Generator
% mode: 1=Training, 2=Inference, 3=Idle
% Output: P_ai_pu (0 to 1), workload_label

workload_label = double(mode);

if mode == 1
    % TRAINING: sustained high with checkpoint dips
    base_power = 0.3;
    checkpoint_interval = 60.0;
    checkpoint_duration = 2.0;
    checkpoint_dip = 0.40;
    comm_period = 1.2;
    comm_amplitude = 0.6;
    
    time_in_cycle = mod(t, checkpoint_interval);
    if time_in_cycle < checkpoint_duration
        P_ai_pu = checkpoint_dip;
    else
        oscillation = comm_amplitude * sin(2.0 * 3.14159 * t / comm_period);
        P_ai_pu = base_power + oscillation;
    end
    
elseif mode == 2
    % INFERENCE: bursty multi-frequency
    base_power = 0.15;
    burst1 = 0.25 * sin(2.0 * 3.14159 * t / 5.0);
    burst2 = 0.15 * sin(2.0 * 3.14159 * t / 1.3);
    burst3 = 0.10 * sin(2.0 * 3.14159 * t / 0.4);
    
    if t < 2.0
        diurnal = 0.5 + 0.5 * (t / 2.0);
    else
        diurnal = 1.0;
    end
    
    P_ai_pu = (base_power + burst1 + burst2 + burst3) * diurnal;
    
elseif mode == 3
    % IDLE
    P_ai_pu = 0.15;
else
    P_ai_pu = 0.5;
end

if P_ai_pu < 0.05
    P_ai_pu = 0.05;
end
if P_ai_pu > 1.0
    P_ai_pu = 1.0;
end

end

== matlab function NE39bus2_PQ/DCLoad4/DC Composite Model/AI Workload Generator ==
  data: t input; mode input; P_ai_pu output; workload_label output
function [P_ai_pu, workload_label] = ai_workload(t, mode)
%#codegen
% AI GPU Workload Profile Generator
% mode: 1=Training, 2=Inference, 3=Idle
% Output: P_ai_pu (0 to 1), workload_label

workload_label = double(mode);

if mode == 1
    % TRAINING: sustained high with checkpoint dips
    base_power = 0.3;
    checkpoint_interval = 60.0;
    checkpoint_duration = 2.0;
    checkpoint_dip = 0.40;
    comm_period = 1.2;
    comm_amplitude = 0.6;
    
    time_in_cycle = mod(t, checkpoint_interval);
    if time_in_cycle < checkpoint_duration
        P_ai_pu = checkpoint_dip;
    else
        oscillation = comm_amplitude * sin(2.0 * 3.14159 * t / comm_period);
        P_ai_pu = base_power + oscillation;
    end
    
elseif mode == 2
    % INFERENCE: bursty multi-frequency
    base_power = 0.15;
    burst1 = 0.25 * sin(2.0 * 3.14159 * t / 5.0);
    burst2 = 0.15 * sin(2.0 * 3.14159 * t / 1.3);
    burst3 = 0.10 * sin(2.0 * 3.14159 * t / 0.4);
    
    if t < 2.0
        diurnal = 0.5 + 0.5 * (t / 2.0);
    else
        diurnal = 1.0;
    end
    
    P_ai_pu = (base_power + burst1 + burst2 + burst3) * diurnal;
    
elseif mode == 3
    % IDLE
    P_ai_pu = 0.15;
else
    P_ai_pu = 0.5;
end

if P_ai_pu < 0.05
    P_ai_pu = 0.05;
end
if P_ai_pu > 1.0
    P_ai_pu = 1.0;
end

end
